simulink model "Compressor_MCU_Simulation_Architecture"  (R2018a)
settings: Solver=FixedStepDiscrete  StartTime=0.0  StopTime=30  FixedStep=TimeSteps.ModelStep  RelTol=1e-6
PreLoadFcn:
  | addpath('tools');
  | addpath('tools\Config_UI');
  | addpath('tools\support');
  | addpath('tools\FMIKit_for_Simulink');
  | addpath('tools\FMIKit_for_Simulink\slx');
  | addpath('tools\SpeedCommand');
  | addpath('tools\SpeedCommand\exe');
  | addpath('tools\SpeedCommand\view');
  | addpath('tools\MciAPI');
  | addpath('tools\MciAPI\exe');
  | addpath('tools\MciAPI\exe\enums');
  | addpath('tools\Read_PDB_File');
  | addpath('tools\Read_PDB_File\exe');
  | addpath('tools\PILComm');
  | addpath('tools\PILComm\exe');
  | 
  | addpath('exe');
  | addpath('source\c_code');
  | addpath('source\simulink\PlantModels\Sensor');
  | addpath('source\simulink\PlantModels\Rectifiers');
  | addpath('source\simulink\PlantModels\Motors\CIM');
  | addpath('source\simulink\PlantModels\Motors\BPM');
  | addpath('source\simulink\PlantModels\Motors\BPM\SFunctions\10k\Dyno');
  | addpath('source\simulink\PlantModels\Motors\BPM\SFunctions\10k\HA');
  | addpath('source\simulink\PlantModels\Motors\BPM\SFunctions\10k\VA_Agitation');
  | addpath('source\simulink\PlantModels\Motors\BPM\SFunctions\10k\VA_Spin');
  | addpath('source\simulink\PlantModels\Motors\BPM\SFunctions\16k\Dyno');
  | addpath('source\simulink\PlantModels\Motors\BPM\SFunctions\16k\HA');
  | addpath('source\simulink\PlantModels\Motors\BPM\SFunctions\16k\VA_Agitation');
  | addpath('source\simulink\PlantModels\Motors\BPM\SFunctions\16k\VA_Spin');
  | addpath('source\simulink\PlantModels\Inverter');
  | addpath('source\simulink\PlantModels\ADCModel');
  | 
  | 
  | addpath('exported_models');
  | clear all;
  | 
  | try
  | FMIKit.initialize()
  | catch
  | display('FMI Kit Initialization Skipped');
  | end
  | 
  | Sim_Arch_Config_UI_App;
PostLoadFcn:
  | myws = get_param(gcs, 'modelworkspace');
  | myws.clear;
  | clear myws;
  | evalin('base', 'recompile_mcu_sim_arch = 1;');
  | updateModelWS(gcs);
  | variant_adc_out_mode = 0;
InitFcn:
  | if (evalin('base', 'exist(''smlarch_need_reset'') == 1'))
  |     msgbox('Reload Variables before Running');
  |     set_param(gcs, 'SimulationCommand', 'stop');
  | end
  | BusInit;
  | if(  (exist('SimArchUID')) && (strcmp(SimArchUID, 'a') == 1)  )
  |     updateModelWS(gcs);
  | end
  | useModelWS(gcs);
  | Simulink.sdi.close;
model workspace (MAT data in the model file):
  DC_Bus.Const_Vbus = 325
  InputCircuit.R_line = 0.8
  InputCircuit.L_line = 5e-05
  InputCircuit.C_buscap = 0.00033
  InputCircuit.R_diode = 0.068
  InputCircuit.R_buscap = 0.603
  InputCircuit.V_knee = 0.75
  InputCircuit.G_off = 1.25e-08
  InputCircuit.L_pfc = 0.0097
  InputCircuit.R_pfc = 0.7
  InputCircuit.Vr = 230
  InputCircuit.Vdc_i = 300
  InputCircuit.freq = 50
  InputCircuit.C1 = -0.200926
  InputCircuit.C2 = 1.64303
  InputCircuit.Cvolt = 0.00738585
  InputCircuit.Vcc = 3.3
  InputCircuit.ADCBit = 12
  InputCircuit.PGA_Gain = 1
  Mechanical.belt_ratio = 10
  Mechanical.JDrum = 0.001
  Mechanical.damp = 0
  Mechanical.m_unb = 0
  Mechanical.r_unb = 0
  Mechanical.M_D = 1
  Mechanical.M = 0.2
  Mechanical.R_Drum = 0.254
  Mechanical.R_J = 0.05
  Mechanical.CF = 0
  Motor.Electrical.Rs_a_Ref = 1.7
  Motor.Electrical.Rs_b_Ref = 1.7
  Motor.Electrical.Rs_c_Ref = 1.7
  Motor.Electrical.p_Pole_Pairs = 3
  Motor.Electrical.PM_Flux_f01 = 0.1273
  Motor.Electrical.PM_Flux_f02 = 0
  Motor.Electrical.PM_Flux_f03 = 0
  Motor.Electrical.PM_Flux_f04 = 0
  Motor.Electrical.PM_Flux_f05 = 0
  Motor.Electrical.PM_Flux_f06 = 0
  Motor.Electrical.PM_Flux_f07 = 0
  Motor.Electrical.PM_Flux_f08 = 0
  Motor.Electrical.PM_Flux_f09 = 0
  Motor.Electrical.PM_Flux_f10 = 0
  Motor.Electrical.PM_Flux_f11 = 0
  Motor.Electrical.PM_Flux_f12 = 0
  Motor.Electrical.PM_Flux_f13 = 0
  Motor.Electrical.ajust = 1.57
  Motor.Electrical.alpha_s = 0.004
  Motor.Mechanical.Jrotor = 0.0002
  Motor.Mechanical.B = 0.002
  Motor.Mechanical.Jadd = 0
  Motor.Mechanical.Rs_Temperature_Ref = 22
  Motor.Mechanical.PM_Temperature_Ref = 22
  Motor.Mechanical.TR = 1
  Motor.Power_Loss.Rot_Loss_Flag = 0
  Motor.Power_Loss.Rot_Loss_Speed0 = 0
  Motor.Power_Loss.Rot_Loss_Speed1 = 500
  Motor.Power_Loss.Rot_Loss_Speed2 = 3000
  Motor.Power_Loss.Rot_Loss_Speed3 = 4000
  Motor.Power_Loss.Rot_Loss_Speed4 = 4000
  Motor.Power_Loss.Rot_Loss_Speed5 = 4000
  Motor.Power_Loss.Rot_Loss_Speed6 = 4000
  Motor.Power_Loss.Rot_Loss_Speed7 = 4000
  Motor.Power_Loss.Rot_Loss_Power0 = 0
  Motor.Power_Loss.Rot_Loss_Power1 = 0
  Motor.Power_Loss.Rot_Loss_Power2 = 0
  Motor.Power_Loss.Rot_Loss_Power3 = 0
  Motor.Power_Loss.Rot_Loss_Power4 = 0
  Motor.Power_Loss.Rot_Loss_Power5 = 0
  Motor.Power_Loss.Rot_Loss_Power6 = 0
  Motor.Power_Loss.Rot_Loss_Power7 = 0
  Motor.Inductance_Variation.Ld_a0 = 0.0205
  Motor.Inductance_Variation.Ld_a1 = 0.0205
  Motor.Inductance_Variation.Ld_a2 = 0.0205
  Motor.Inductance_Variation.Ld_a3 = 0.0205
  Motor.Inductance_Variation.Ld_a4 = 0.0205
  Motor.Inductance_Variation.Ld_a5 = 0.0205
  Motor.Inductance_Variation.Ld_a6 = 0.0205
  Motor.Inductance_Variation.Ld_a7 = 0.0205
  Motor.Inductance_Variation.Lq_b0 = 0.0205
  Motor.Inductance_Variation.Lq_b1 = 0.0205
  Motor.Inductance_Variation.Lq_b2 = 0.0205
  Motor.Inductance_Variation.Lq_b3 = 0.0205
  Motor.Inductance_Variation.Lq_b4 = 0.0205
  Motor.Inductance_Variation.Lq_b5 = 0.0205
  Motor.Inductance_Variation.Lq_b6 = 0.0205
  Motor.Inductance_Variation.Lq_b7 = 0.0205
  Motor.Inductance_Variation.I_pk0 = 0
  Motor.Inductance_Variation.I_pk1 = 1
  Motor.Inductance_Variation.I_pk2 = 2
  Motor.Inductance_Variation.I_pk3 = 3
  Motor.Inductance_Variation.I_pk4 = 4
  Motor.Inductance_Variation.I_pk5 = 5
  Motor.Inductance_Variation.I_pk6 = 6
  Motor.Inductance_Variation.I_pk7 = 7
  Paths.complete_file_R = 'settings\ParametersFiles\Rectifier_Parameters\HVPS_230VPFC\WindyStripH50_AC230VPFC.xml'
  Paths.complete_file_M = 'settings\ParametersFiles\Motor_Parameters\BPM\sBPM\BPM_RECHI_Heatpump.xml'
  Paths.complete_file_mc = 'settings\ParametersFiles\Mechanical_Parameters\HA\Mechanical_HA.xml'
  Paths.chosen_dir_M = 'settings\ParametersFiles\Motor_Parameters\BPM\sBPM'
  Paths.Setting_File_Path = 'C:\Data\Prj2021\Mcu_FOC_Control_Vcc_Dryer\exe\settingfile.bin'
  Paths.Root_Path = 'C:\Data\Prj2021\Mcu_FOC_Control_Vcc_Dryer\source'
  Paths.Object_Path = ''
  Thermal.Tstator = 22
  Thermal.Trotor = 22
  TimeSteps.ModelStep = 0.0001
  TimeSteps.InputCircuitStep = 0.0005
  Variant_Input_Circuit = 5
  Variant_Motor = 3
  Variant_Motor_Control = 1
  Variant_Sensor = 0
  config.MCI_Sampling_Frequency = 'Set'
  config.rect_flag = 0
  config.const_dcbus_flag = 1
  config.Root_Path_flag = 'Source Selected'
  config.Motor_Control_Source = 'Set'
  config.Control_Layer = 'SIL'
  config.Fast_ADC_Initialization_Flag = 'Set'
  config.Skip_Motor_Moving_Handler_Flag = 'Set'
  config.BoardVariant = 'AC230VPFC'
  config.MotorVariant = 'BPM_RECHI_Heatpump'
  config.MechanicalVariant = 'DynoLoad'
  config.Setting_File_Flag = 'Set'
undefined symbols (not defined in the file): sigbuilder_block, steps
libraries: pdb_libbrowser x6, mciapi_libbrowser x1
CloseFcn:
  | rmpath('support');
  | rmpath('Compile Scripts');
  | rmpath(genpath('Plant Models'));
  | rmpath(genpath('MciAPI'));
  | clc;
  | clear all;
settings Model: Creator=consul.marchionne  LastModifiedBy=BEATOA
settings DataIOCC: LimitDataPoints=on
settings OptimizationCC: LifeSpan=inf
settings DebuggingCC: SolverPrmCheckMsg=warning  SFUnexpectedBacktrackingDiag=warning  SFNoUnconditionalDefaultTransitionDiag=warning  SFExecutionAtInitializationDiag=none
settings HardwareCC: ProdBitPerPointer=32  ProdBitPerSizeT=32  ProdBitPerPtrDiffT=32  ProdLargestAtomicFloat=None  ProdIntDivRoundTo=Undefined  ProdEndianess=Unspecified  ProdWordSize=32  ProdHWDeviceType=32-bit Generic
settings ModelReferenceCC: UpdateModelReferenceTargets=IfOutOfDate  EnableRefExpFcnMdlSchedulingChecks=off  ModelReferenceNumInstancesAllowed=Single  ModelReferenceMinAlgLoopOccurrences=on  PropagateSignalLabelsOutOfModel=off
settings CodeAppCC: StateflowObjectComments=on
settings GRTTargetCC: TargetLangStandard=C89/C90 (ANSI)  GeneratePreprocessorConditionals=Disable all
settings ConfigComp: CovMetricSettings=dw  CovHtmlReporting=on  CovSaveCumulativeToWorkspaceVar=on  CovSaveSingleToWorkspaceVar=on  CovExternalEMLEnable=off  CovSFcnEnable=off

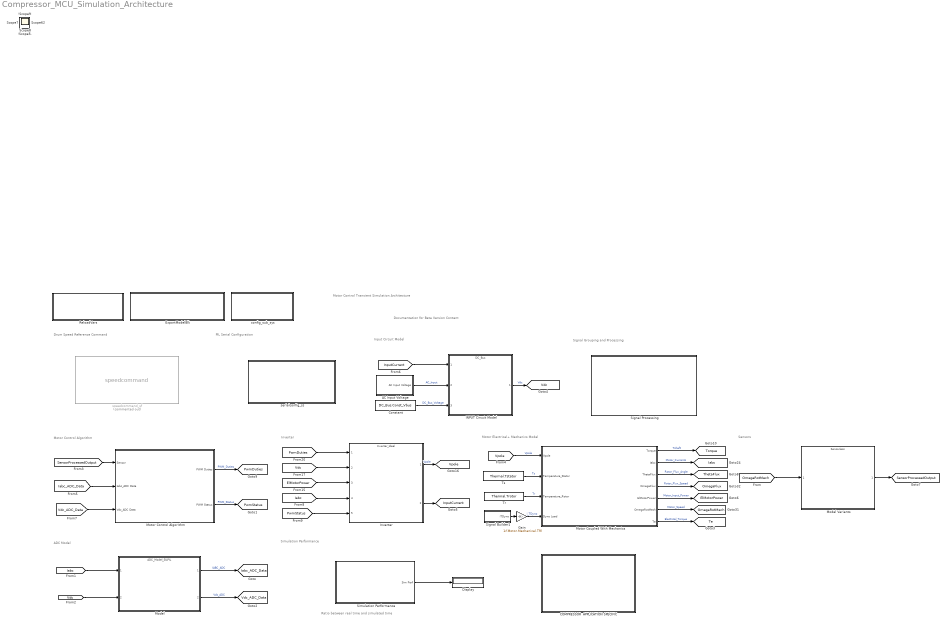
== system Compressor_MCU_Simulation_Architecture ==
  note: Motor Control Transient Simulation Architecture
  note: Input Circuit Model
  note: Simulation Performance
  note: Ratio between real time and simulated time
  note: ADC Model
  note: Motor Electrical+ Mechanics Model
  note: Inverter
  note: Signal Grouping and Processing
  note: PIL Serial Configuration
  note: Motor Control Algorithm
  note: Sensors
  note: Drum Speed Reference Command
  note: Documentation for Beta Version Content
  AC Input Voltage : Subsystem
  COMPRESSOR  APPLICATION SPECIFIC : Subsystem
  Constant : Constant  Value=DC_Bus.Const_Vbus
  Display : Display
  ExportModelBlk : Subsystem  LoadFcn=|  mask{model_name=}
      | msk = Simulink.Mask.get(gcb);
      | bHandle = msk.getDialogControl('Control2');
      | bHandle.Enabled = 'on';
      | clear msk;
      | clear bHandle;
      mask prompts: model_name "Model's export name (no extension)"
      mask DialogControl Control2 Prompt: Export
      mask DialogControl Control2 Callback:
      | save_system('MCU_Simulation_Architecture');
      | if (strcmp(get_param(gcb, 'model_name'),'') == 1)
      |     msgbox('Must give a name to the model');
      | else
      |     exportSimArch(get_param(gcb, 'model_name'));
      | end
      mask Display: disp('Export current configuration');
  Gain : Gain  Gain=1/(Motor.Mechanical.TR)
  INPUT Circuit Model : ModelReference  ModelNameDialog=DC_Bus.slx  SimulationMode=Normal  Variant=on  ModelReferenceVersion=1.7
      settings: AttributesFormatString=%<ActiveVariant>
  Inverter : ModelReference  ModelNameDialog=Inverter_Ideal.slx  SimulationMode=Normal  Variant=on  OverrideUsingVariant=Variant1  ModelReferenceVersion=1.14
      settings: AttributesFormatString=%<ActiveVariant>
  Model : ModelReference  ModelNameDialog=ADC_Model_SILPIL.slx  SimulationMode=Normal  ModelReferenceVersion=1.7
  Model Variants : ModelReference  ModelNameDialog=Sensorless.slx  SimulationMode=Normal  Variant=on  ModelReferenceVersion=1.8
      settings: AttributesFormatString=%<ActiveVariant>
  Motor Control Algorithm : Subsystem  SystemSampleTime=6.25e-5
  Motor Coupled With Mechanics : Subsystem  SystemSampleTime=0.000125
      settings: CopyFcn=|
      | blockname = gcb;
      |  linkstatus = lower(get_param(blockname,'LinkStatus'));
      | if strcmp(linkstatus,'resolved')
      |   set_param(gcb,'LinkStatus','none');
      | end
  ReloadVars : Subsystem
      settings: OpenFcn=|
      | evalin('base', 'clear smlarch_need_reset');
      | useModelWS(gcs);
      mask Display: disp('Reload Variables');
  Signal Builder1 : Subsystem  Tag=STV Subsys  LoadFcn=sigbuilder_block('load');  StartFcn=sigbuilder_block('start');  StopFcn=sigbuilder_block('stop');  ClipboardFcn=sigbuilder_block('clipboard');  mask(Sigbuilder block){tuvar=[0:10]}
      mask help: Simulink:masks:SigbuilderBlock_MD
      mask init:
      | if ~strcmp(get_param(bdroot(gcbh),'SimulationStatus'),'stopped') tuvar = sigbuilder_block('maskInit'); end
      settings: CopyFcn=sigbuilder_block('copy');  DeleteFcn=sigbuilder_block('delete');  ModelCloseFcn=sigbuilder_block('modelClose');  PreSaveFcn=sigbuilder_block('preSave');  PauseFcn=sigbuilder_block('pause');  ContinueFcn=sigbuilder_block('continue');  NameChangeFcn=sigbuilder_block('namechange');  OpenFcn=sigbuilder_block('open',[150 123 461.25 300 ]);  CloseFcn=sigbuilder_block('close');
      mask Display: plot(0, 0, 100, 100,[2, 2, 32, 32, 2], [68, 8, 8, 68, 68],[32, 2], [38, 38], [32, 19, 2],[53, 60, 44], [32, 17, 17, 2],[16, 16, 31, 31]);txt = getActiveGroup(gcbh);text(2, 100, txt,'verticalAlignment', 'top');
  Signal Processing : Subsystem
  Simulation Performance : Subsystem
  Tr : Constant  Value=Thermal.Trotor
  Ts : Constant  Value=Thermal.Tstator
  config_sub_sys : Subsystem  TreatAsAtomicUnit=on  mask{mcu_recompile=on}
      mask prompts: mcu_recompile "Recompile"
      mask Display:
      | if (strcmp(get_param(gcb, 'mcu_recompile'),'off') == 1)
      |     disp('Do not Recompile');
      | else
      |     disp('Recompile');
      | end
  serialconfig_ss : Subsystem  mask{comdevtype=RS232, com_port=COM4, baudrate=57600}
      mask prompts: comdevtype "COM Type"; com_port "COM Port"
      mask TypeOptions comdevtype: RS232 | SPI
      mask Callback comdevtype:
      | maskStr = get_param(gcb,'comdevtype');
      | if strcmp(maskStr,'SPI')
      |     assignin('base', 'VARIANT_PIL_COMM', 2);
      | else
      |     assignin('base', 'VARIANT_PIL_COMM', 1);
      | end
      | clear maskStr;
      mask TypeOptions com_port: COM3 | COM4
      mask TypeOptions baudrate: 2400 | 4800 | 9600 | 19200 | 28800 | 38400 | 57600 | 115200 | 230400
      mask DialogControl ParameterGroupVar Prompt: RS232 Settings
      mask DialogControl rfrsh_button Prompt: Refresh Ports
      mask DialogControl rfrsh_button Callback:
      | devices = winqueryreg('name', 'HKEY_LOCAL_MACHINE', 'HARDWARE\DEVICEMAP\SERIALCOMM');
      | if (isempty(devices))
      |     com{1} = 'NONE';
      | else
      |     com = cell(1, length(devices));
      |    % h = waitbar(0,'Scanning Serial Ports...','Name','Scanning Serial Ports...');
      |     for i = 1:length(devices)
      |         com{i} = winqueryreg('HKEY_LOCAL_MACHINE', 'HARDWARE\DEVICEMAP\SERIALCOMM', devices{i});
      |     %    waitbar(i/length(devices),h);
      |     end
      | end
      | 
      | msk = Simulink.Mask.get(gcb);
      | p = msk.Parameters;
      | p(2).TypeOptions = com;
      | clear msk;
      | clear p;
      | clear com;
      | clear devices;
      mask Display: disp('Serial Configuration');
  speedcommand_sf : S-Function  Commented=on  InitFcn=|  StopFcn=|  FunctionName=speedcommand  Parameters=steps, Variant_Motor_Control  SFunctionDeploymentMode=off  EnableBusSupport=off
      InitFcn=|
      | transmission = evalin('base','Motor.Mechanical.TR');
      | if isempty(get_param(gcb,'UserData'))
      | steps = [];
      | else
      |     ud = get_param(gcb,'UserData');
      |     [pts,steps] = GenPlotCmds(ud.table);
      |     for i = 1:size(steps,1)
      |         steps(i,1) = steps(i,1) * transmission;
      |         steps(i,2) = steps(i,2) * transmission;
      |     end
      | end
      | clear transmission;
      | clear i;
      | clear ud;
      StopFcn=|
      | clear steps;
      | clear pts;
      settings: OpenFcn=SpeedCommandView;
  Scope{,2..12} (12 alike) : Scope
  tag scope: ElMotorPower=global, Iabc=global, Iabc_ADC_Data=global, InputCurrent=global, OmegaFlux=global, OmegaRotMech=global, PwmDuties=global, PwmStatus=global, SensorProcessedOutput=global, Te=global, ThetaFlux=global, Torque=global, Vdc=global, Vdc_ADC_Data=global, Vpole=global
  wires:
  [OmegaRotMech] -> Model Variants/1
  Simulation Performance/1(Sim Perf) -> Display/1
  [Vpole] -> Motor Coupled With Mechanics/1(Vpole)  "Vpole"
  Motor Coupled With Mechanics/1(Torque) -> [Torque]  "Tshaft"
  Motor Coupled With Mechanics/2(Iabc) -> [Iabc]  "Motor_Currents"
  Motor Coupled With Mechanics/3(ThetaFlux) -> [ThetaFlux]  "Rotor_Flux_Angle"
  Motor Coupled With Mechanics/4(OmegaFlux) -> [OmegaFlux]  "Rotor_Flux_Speed"
  Motor Coupled With Mechanics/5(ElMotorPower) -> [ElMotorPower]  "Motor_Input_Power"
  Motor Coupled With Mechanics/6(OmegaRotMech) -> [OmegaRotMech]  "Motor_Speed"
  [PwmDuties] -> Inverter/1
  [Vdc] -> Inverter/2
  [ElMotorPower] -> Inverter/3
  [Iabc] -> Inverter/4
  Inverter/1 -> [Vpole]  "Vpole"
  Inverter/2 -> [InputCurrent]
  Motor Control Algorithm/1(PWM Duties) -> [PwmDuties]  "PWM_Duties"
  Motor Control Algorithm/2(PWM Status) -> [PwmStatus]  "PWM_Status"
  [SensorProcessedOutput] -> Motor Control Algorithm/1(Sensor)
  INPUT Circuit Model/1 -> [Vdc]  "Vdc"
  Constant/1 -> INPUT Circuit Model/3  "DC_Bus_Voltage"
  AC Input Voltage/1(AC Input Voltage) -> INPUT Circuit Model/2  "AC_Input"
  [InputCurrent] -> INPUT Circuit Model/1
  Model Variants/1 -> [SensorProcessedOutput]
  [PwmStatus] -> Inverter/5
  [Vdc] -> Model/2
  [Iabc] -> Model/1
  [Iabc_ADC_Data] -> Motor Control Algorithm/2(Iabc_ADC Data)
  Model/1 -> [Iabc_ADC_Data]  "IABC_ADC"
  Model/2 -> [Vdc_ADC_Data]  "Vdc_ADC"
  [Vdc_ADC_Data] -> Motor Control Algorithm/3(Vdc_ADC Data)
  Ts/1 -> Motor Coupled With Mechanics/2(Temperature_Stator)  "Ts"
  Tr/1 -> Motor Coupled With Mechanics/3(Temperature_Rotor)  "Tr"
  Gain/1 -> Motor Coupled With Mechanics/4(Dyno Load)  "i_TDyno"
  Signal Builder1/1(iTDyno) -> Gain/1
  Motor Coupled With Mechanics/7(Te) -> [Te]  "Electrical_Torque"

== system Compressor_MCU_Simulation_Architecture/AC Input Voltage ==
  Sine Wave : Sin  Amplitude=InputCircuit.Vr*sqrt(2)  Frequency=InputCircuit.freq*2*pi
  AC Input Voltage : Outport
  wires:
  Sine Wave/1 -> AC Input Voltage/1

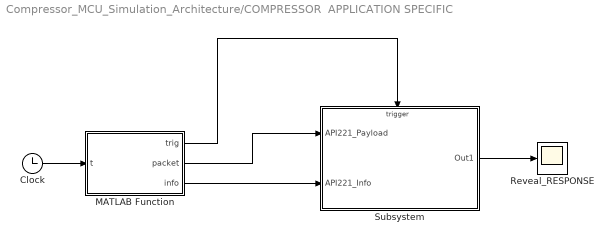
== system Compressor_MCU_Simulation_Architecture/COMPRESSOR  APPLICATION SPECIFIC ==
  Clock : Clock
  MATLAB Function : MATLAB Function  TreatAsAtomicUnit=on
  Reveal_RESPONSE : Scope
  Subsystem : Subsystem
  wires:
  MATLAB Function/1(trig) -> Subsystem/Trigger
  MATLAB Function/2(packet) -> Subsystem/1(API221_Payload)
  Clock/1 -> MATLAB Function/1(t)
  Subsystem/1(Out1) -> Reveal_RESPONSE/1
  MATLAB Function/3(info) -> Subsystem/2(API221_Info)

== system Compressor_MCU_Simulation_Architecture/ExportModelBlk ==

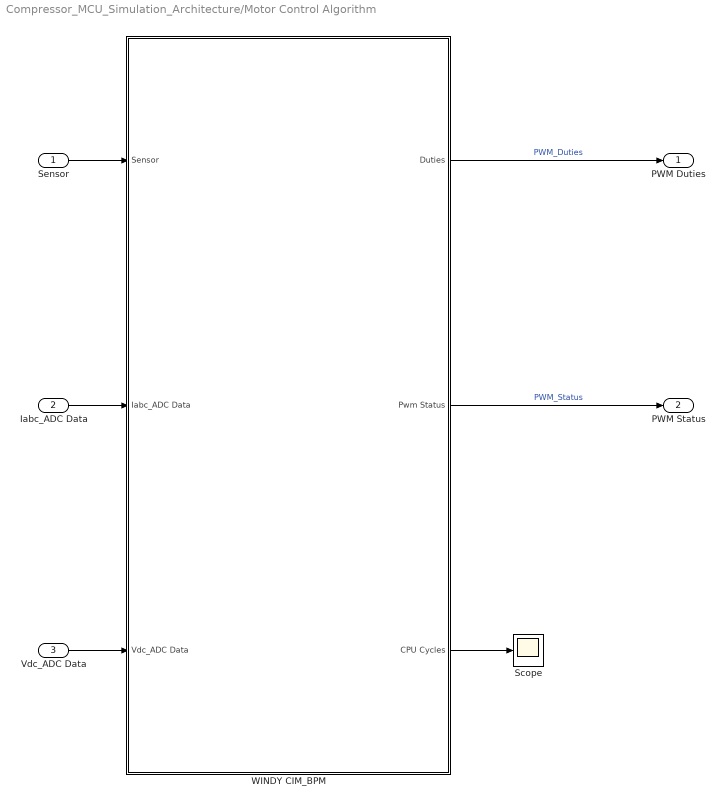
== system Compressor_MCU_Simulation_Architecture/Motor Control Algorithm ==
  Sensor : Inport
  Iabc_ADC Data : Inport  Port=2
  Vdc_ADC Data : Inport  Port=3
  Scope : Scope
  WINDY CIM_BPM : Subsystem  Variant=on
  PWM Duties : Outport
  PWM Status : Outport  Port=2
  wires:
  WINDY CIM_BPM/1(Duties) -> PWM Duties/1  "PWM_Duties"
  WINDY CIM_BPM/2(Pwm Status) -> PWM Status/1  "PWM_Status"
  Sensor/1 -> WINDY CIM_BPM/1(Sensor)
  Iabc_ADC Data/1 -> WINDY CIM_BPM/2(Iabc_ADC Data)
  Vdc_ADC Data/1 -> WINDY CIM_BPM/3(Vdc_ADC Data)
  WINDY CIM_BPM/3(CPU Cycles) -> Scope/1

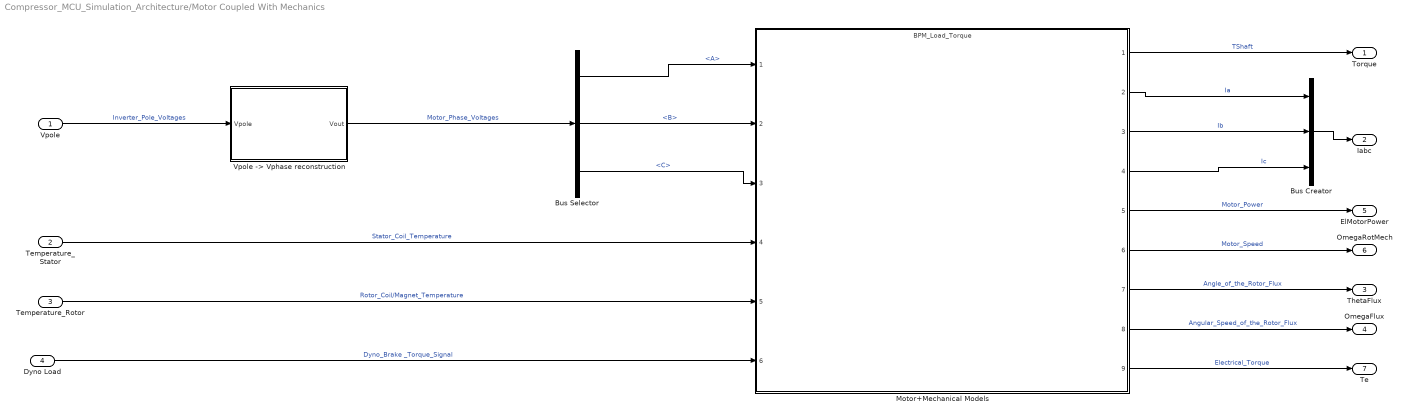
== system Compressor_MCU_Simulation_Architecture/Motor Coupled With Mechanics ==
  Vpole : Inport  OutDataTypeStr=Bus: XabcBus
  Temperature_Stator : Inport  Port=2
  Temperature_Rotor : Inport  Port=3
  Dyno Load : Inport  Port=4
  Bus Creator : BusCreator  Inputs=3
  Bus Selector : BusSelector  OutputSignals=A,B,C
  Motor+Mechanical Models : ModelReference  ModelNameDialog=BPM_Load_Torque.slx  SimulationMode=Normal  Variant=on  ModelReferenceVersion=1.264
      settings: AttributesFormatString=%<ActiveVariant>
  "Vpole -> Vphase reconstruction" : MATLAB Function  TreatAsAtomicUnit=on
  Torque : Outport
  Iabc : Outport  Port=2  OutDataTypeStr=Bus: XabcBus
  ThetaFlux : Outport  Port=3
  OmegaFlux : Outport  Port=4
  ElMotorPower : Outport  Port=5
  OmegaRotMech : Outport  Port=6
  Te : Outport  Port=7
  wires:
  Bus Creator/1 -> Iabc/1
  Vpole/1 -> "Vpole -> Vphase reconstruction"/1(Vpole)  "Inverter_Pole_Voltages"
  "Vpole -> Vphase reconstruction"/1(Vout) -> Bus Selector/1  "Motor_Phase_Voltages"
  Bus Selector/1 -> Motor+Mechanical Models/1  "<A>"
  Bus Selector/2 -> Motor+Mechanical Models/2  "<B>"
  Bus Selector/3 -> Motor+Mechanical Models/3  "<C>"
  Temperature_Stator/1 -> Motor+Mechanical Models/4  "Stator_Coil_Temperature"
  Temperature_Rotor/1 -> Motor+Mechanical Models/5  "Rotor_Coil/Magnet_Temperature"
  Motor+Mechanical Models/1 -> Torque/1  "TShaft"
  Motor+Mechanical Models/2 -> Bus Creator/1  "Ia"
  Motor+Mechanical Models/3 -> Bus Creator/2  "Ib"
  Motor+Mechanical Models/4 -> Bus Creator/3  "Ic"
  Motor+Mechanical Models/5 -> ElMotorPower/1  "Motor_Power"
  Motor+Mechanical Models/6 -> OmegaRotMech/1  "Motor_Speed"
  Motor+Mechanical Models/7 -> ThetaFlux/1  "Angle_of_the_Rotor_Flux"
  Dyno Load/1 -> Motor+Mechanical Models/6  "Dyno_Brake _Torque_Signal"
  Motor+Mechanical Models/8 -> OmegaFlux/1  "Angular_Speed_of_the_Rotor_Flux"
  Motor+Mechanical Models/9 -> Te/1  "Electrical_Torque"

== system Compressor_MCU_Simulation_Architecture/ReloadVars ==

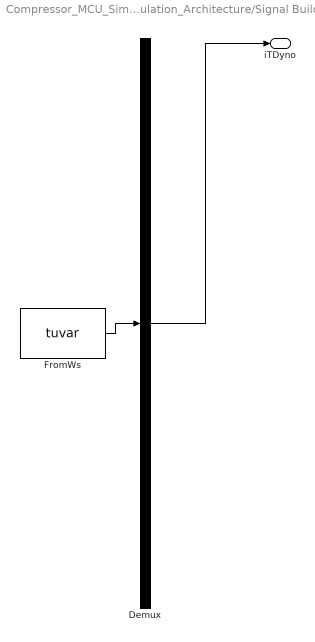
== system Compressor_MCU_Simulation_Architecture/Signal Builder1 ==
  Demux : Demux  Tag=STV Demux  Outputs=1
  FromWs : FromWorkspace  Tag=STV FromWs  VariableName=tuvar  SampleTime=0
      SigBuilderData=|
      | common.afterFinalStr = 'Extrapolate'
      | common.sampleTime = 0
      | dataSet.timeRange = [0 30]
      | dataSet.name = 'Dyno_Load_Profile'
      | sbobj.Groups.Name = 'Dyno_Load_Profile'
      | sbobj.Groups.Signals.Name = 'iTDyno'
      | sbobj.Groups.Signals.XData = [0 0.8 4 20 28 30]
      | sbobj.Groups.Signals.YData = [0 0 0 0 0 0]
      | sbobj.Groups.TimeRange = [0 30]
  iTDyno : Outport  Tag=STV Outport
  wires:
  Demux/1 -> iTDyno/1
  FromWs/1 -> Demux/1

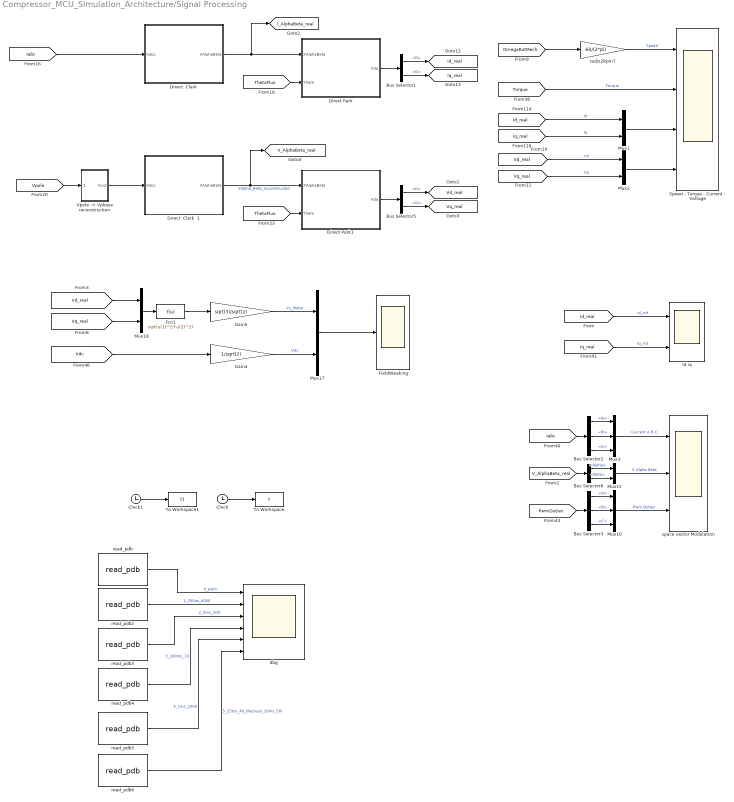
== system Compressor_MCU_Simulation_Architecture/Signal Processing ==
  Bus Selector1 : BusSelector  OutputSignals=D,Q
  Bus Selector2 : BusSelector  OutputSignals=Ia,Ib,Ic
  Bus Selector3 : BusSelector  OutputSignals=A,B,C
  Bus Selector5 : BusSelector  OutputSignals=D,Q
  Bus Selector6 : BusSelector  OutputSignals=Alpha,Beta
  Clock : Clock
  Clock1 : Clock
  "Direct  Clark  " : MATLAB Function  TreatAsAtomicUnit=on  SystemSampleTime=SystemSampleTime  mask{SystemSampleTime=-1}
      mask prompts: SystemSampleTime "Simulink:blkprm_prompts:AllBlksSampleTime"
  Direct  Clark  1 : MATLAB Function  TreatAsAtomicUnit=on  SystemSampleTime=SystemSampleTime  mask{SystemSampleTime=-1}
      mask prompts: SystemSampleTime "Simulink:blkprm_prompts:AllBlksSampleTime"
  Direct Park : MATLAB Function  TreatAsAtomicUnit=on  SystemSampleTime=SystemSampleTime  mask{SystemSampleTime=-1}
      mask prompts: SystemSampleTime "Simulink:blkprm_prompts:AllBlksSampleTime"
  Direct Park1 : MATLAB Function  TreatAsAtomicUnit=on  SystemSampleTime=SystemSampleTime  mask{SystemSampleTime=-1}
      mask prompts: SystemSampleTime "Simulink:blkprm_prompts:AllBlksSampleTime"
  Fcn1 : Fcn  Expr=sqrt(u(1)^2+u(2)^2)
  "FieldWeaking " : Scope
  Gain4 : Gain  Gain=1/sqrt(2)
  Gain5 : Gain  Gain=sqrt(3)/sqrt(2)
  Id iq : Scope  NumInputPorts=2
  Mux{1..2,15,17..18} (5 alike) : Mux  Inputs=2
  Mux10 : Mux  Inputs=3
  Mux3 : Mux  Inputs=3
  Speed - Torque - Current - Voltage : Scope  NumInputPorts=4
  To Workspace : ToWorkspace  VariableName=t  SampleTime=-1
      settings: Save2DSignal=2-D array (concatenate along first dimension)
  To Workspace1 : ToWorkspace  VariableName=t1  SampleTime=-1
      settings: Save2DSignal=2-D array (concatenate along first dimension)
  "Vpole -> Vphase reconstruction" : MATLAB Function  TreatAsAtomicUnit=on
  dbg : Scope  NumInputPorts=6
  rad/s2Rpm7 : Gain  Gain=60/(2*pi)
  read_pdb : pdb_libbrowser/read_pdb  vstring=dbg_scheduler_0
      settings: SourceProductName=Sim Arch
  read_pdb2 : pdb_libbrowser/read_pdb  vstring=dbg_scheduler_1
      settings: SourceProductName=Sim Arch
  read_pdb3 : pdb_libbrowser/read_pdb  vstring=dbg_scheduler_2
      settings: SourceProductName=Sim Arch
  read_pdb4 : pdb_libbrowser/read_pdb  vstring=dbg_scheduler_3
      settings: SourceProductName=Sim Arch
  read_pdb5 : pdb_libbrowser/read_pdb  vstring=dbg_scheduler_4
      settings: SourceProductName=Sim Arch
  read_pdb6 : pdb_libbrowser/read_pdb  vstring=dbg_scheduler_5
      settings: SourceProductName=Sim Arch
  space vector Modulation : Scope  NumInputPorts=3
  tag scope: I_AlphaBeta_real=global, Id_real=global, Iq_real=global, V_AlphaBeta_real=global, Vd_real=global, Vq_real=global
  wires:
  [OmegaRotMech] -> rad/s2Rpm7/1
  rad/s2Rpm7/1 -> Speed - Torque - Current - Voltage/1  "Speed"
  [Vq_real] -> Mux2/2  "Vq"
  [Id_real] -> Mux1/1  "Id"
  [Iabc] -> "Direct  Clark  "/1(Xabc)
  Direct Park/1(Xdq) -> Bus Selector1/1
  Bus Selector1/1 -> [Id_real]  "<D>"
  Bus Selector1/2 -> [Iq_real]  "<Q>"
  Fcn1/1 -> Gain5/1
  Mux18/1 -> Fcn1/1
  [Vd_real] -> Mux18/1
  [Vq_real] -> Mux18/2
  Mux17/1 -> "FieldWeaking "/1
  [Vdc] -> Gain4/1
  Bus Selector3/1 -> Mux10/1  "<A>"
  Bus Selector3/2 -> Mux10/2  "<B>"
  Bus Selector3/3 -> Mux10/3  "<C>"
  Mux10/1 -> space vector Modulation/3  "Pwm Duties"
  Bus Selector2/1 -> Mux3/1  "<Ia>"
  Bus Selector2/2 -> Mux3/2  "<Ib>"
  Bus Selector2/3 -> Mux3/3  "<Ic>"
  [Iabc] -> Bus Selector2/1
  [PwmDuties] -> Bus Selector3/1
  "Direct  Clark  "/1(XAlphaBeta) -> [I_AlphaBeta_real], Direct Park/1(XAlphaBeta)
  Clock/1 -> To Workspace/1
  Clock1/1 -> To Workspace1/1
  [Id_real] -> Id iq/1  "Id_rot"
  [Iq_real] -> Id iq/2  "Iq_rot"
  Gain4/1 -> Mux17/2  "Vdc"
  Gain5/1 -> Mux17/1  "Vs_Motor"
  Mux3/1 -> space vector Modulation/1  "Current A B C"
  [ThetaFlux] -> Direct Park/2(Theta)
  "Vpole -> Vphase reconstruction"/1(Vout) -> Direct  Clark  1/1(Xabc)
  [Vpole] -> "Vpole -> Vphase reconstruction"/1(Vpole)
  Direct  Clark  1/1(XAlphaBeta) -> Direct Park1/1(XAlphaBeta), [V_AlphaBeta_real]  "Valpha_Beta_reconstructed"
  [V_AlphaBeta_real] -> Bus Selector6/1
  Bus Selector6/1 -> Mux15/1  "<Alpha>"
  Bus Selector6/2 -> Mux15/2  "<Beta>"
  Mux15/1 -> space vector Modulation/2  "V Alpha Beta"
  Bus Selector5/2 -> [Vq_real]  "<Q>"
  Bus Selector5/1 -> [Vd_real]  "<D>"
  [ThetaFlux] -> Direct Park1/2(Theta)
  Direct Park1/1(Xdq) -> Bus Selector5/1
  [Iq_real] -> Mux1/2  "Iq"
  [Vd_real] -> Mux2/1  "Vd"
  [Torque] -> Speed - Torque - Current - Voltage/2  "Torque"
  Mux2/1 -> Speed - Torque - Current - Voltage/4
  Mux1/1 -> Speed - Torque - Current - Voltage/3
  read_pdb4/1 -> dbg/4  "3_100ms_10"
  read_pdb6/1 -> dbg/6  "5_25ms_40_(Nucleus_20ms_50)"
  read_pdb3/1 -> dbg/3  "2_5ms_200"
  read_pdb5/1 -> dbg/5  "4_1ms_1000"
  read_pdb2/1 -> dbg/2  "1_250us_4000"
  read_pdb/1 -> dbg/1  "0_pwm"

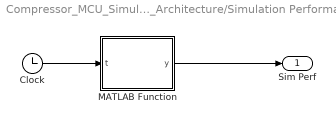
== system Compressor_MCU_Simulation_Architecture/Simulation Performance ==
  Clock : Clock
  MATLAB Function : MATLAB Function  TreatAsAtomicUnit=on
  Sim Perf : Outport
  wires:
  MATLAB Function/1(y) -> Sim Perf/1
  Clock/1 -> MATLAB Function/1(t)

== system Compressor_MCU_Simulation_Architecture/config_sub_sys ==

== system Compressor_MCU_Simulation_Architecture/serialconfig_ss ==

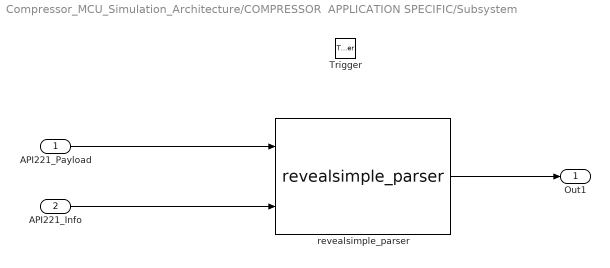
== system Compressor_MCU_Simulation_Architecture/COMPRESSOR  APPLICATION SPECIFIC/Subsystem ==
  API221_Payload : Inport
  API221_Info : Inport  Port=2
  Trigger : TriggerPort  VariantControl=Variant  PortDimensions=1
  revealsimple_parser : mciapi_libbrowser/revealsimple_parser  SFunctionModules=''
      settings: SourceProductName=Sim Arch
  Out1 : Outport
  wires:
  revealsimple_parser/1 -> Out1/1
  API221_Payload/1 -> revealsimple_parser/1
  API221_Info/1 -> revealsimple_parser/2

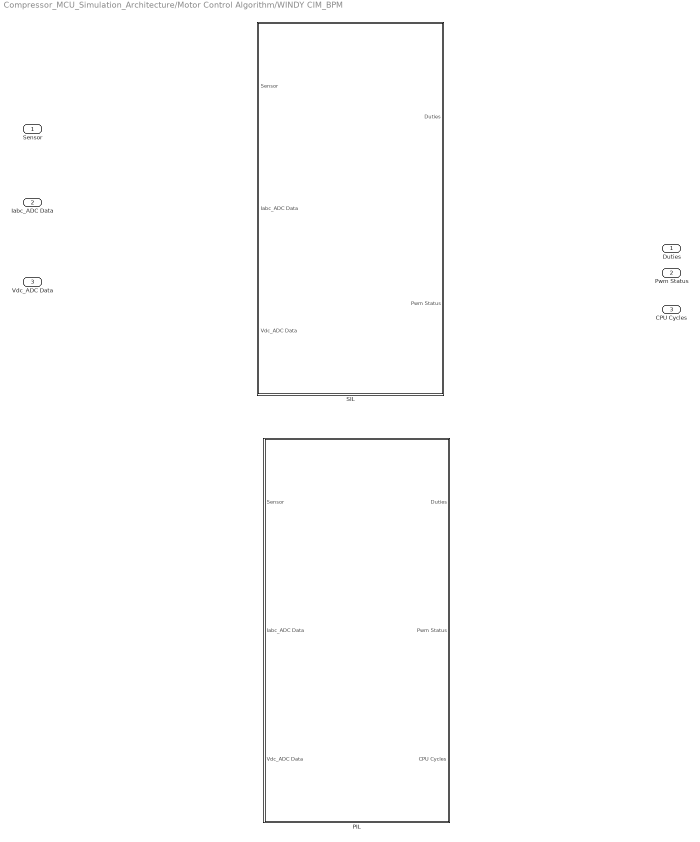
== system Compressor_MCU_Simulation_Architecture/Motor Control Algorithm/WINDY CIM_BPM ==
  Sensor : Inport
  Iabc_ADC Data : Inport  Port=2
  Vdc_ADC Data : Inport  Port=3
  PIL : Subsystem  InitFcn=|  VariantControl=Variant_Motor_Control==2
      | Control_Layer=evalin('base','config.Control_Layer');
      | 
      | switch Control_Layer
      |    case 'MCI'
      | 
      |      Compile_Link_MCI(config.Root_Path_flag, Paths.Root_Path, config.Motor, Paths.Object_Path)
      | 
      | case 'MCU'
      |    
      |      Compile_Link_MCU(config.Root_Path_flag, Paths.Root_Path, config.Motor, Paths.Object_Path)
      | end
      | 
      | clear Control_Layer;
  SIL : Subsystem  VariantControl=Variant_Motor_Control==1
  Duties : Outport
  Pwm Status : Outport  Port=2
  CPU Cycles : Outport  Port=3

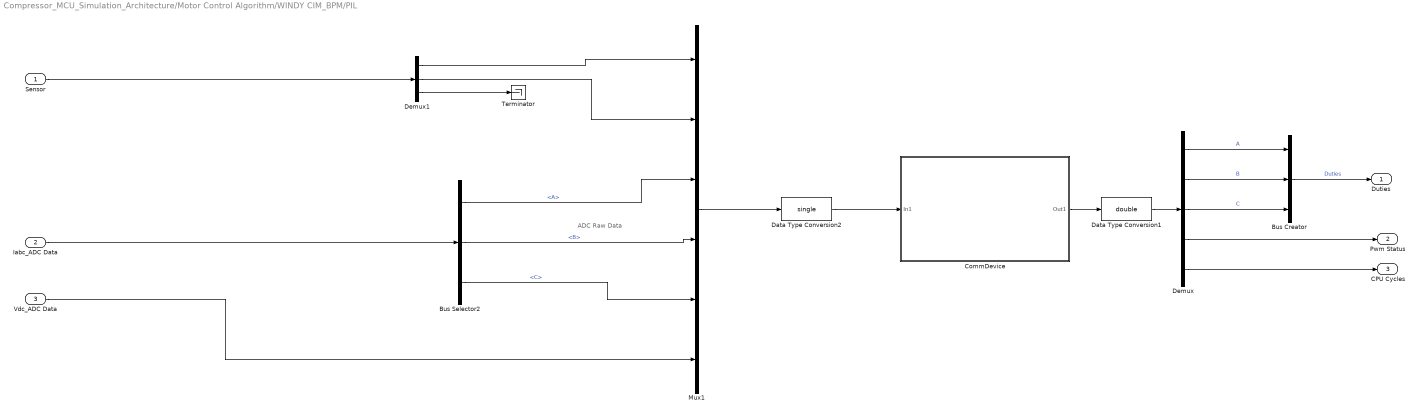
== system Compressor_MCU_Simulation_Architecture/Motor Control Algorithm/WINDY CIM_BPM/PIL ==
  note: ADC Raw Data
  Sensor : Inport
  Iabc_ADC Data : Inport  Port=2
  Vdc_ADC Data : Inport  Port=3
  Bus Creator : BusCreator  Inputs=3
  Bus Selector2 : BusSelector  OutputSignals=A,B,C
  CommDevice : Subsystem  Variant=on  VariantControl=Variant1
  Data Type Conversion1 : DataTypeConversion  OutDataTypeStr=double
  Data Type Conversion2 : DataTypeConversion  OutDataTypeStr=single
  Demux : Demux  Outputs=5
  Demux1 : Demux  Outputs=3
  Mux1 : Mux  Inputs=6
  Terminator : Terminator
  Duties : Outport
  Pwm Status : Outport  Port=2
  CPU Cycles : Outport  Port=3
  wires:
  Bus Creator/1 -> Duties/1  "Duties"
  Bus Selector2/2 -> Mux1/4  "<B>"
  Bus Selector2/1 -> Mux1/3  "<A>"
  Bus Selector2/3 -> Mux1/5  "<C>"
  Vdc_ADC Data/1 -> Mux1/6
  Iabc_ADC Data/1 -> Bus Selector2/1
  Sensor/1 -> Demux1/1
  Demux1/3 -> Terminator/1
  Demux1/1 -> Mux1/1
  Demux1/2 -> Mux1/2
  Mux1/1 -> Data Type Conversion2/1
  Data Type Conversion2/1 -> CommDevice/1("In1 ")
  Data Type Conversion1/1 -> Demux/1
  Demux/4 -> Pwm Status/1
  Demux/1 -> Bus Creator/1  "A"
  Demux/2 -> Bus Creator/2  "B"
  Demux/3 -> Bus Creator/3  "C"
  CommDevice/1(" Out1") -> Data Type Conversion1/1
  Demux/5 -> CPU Cycles/1

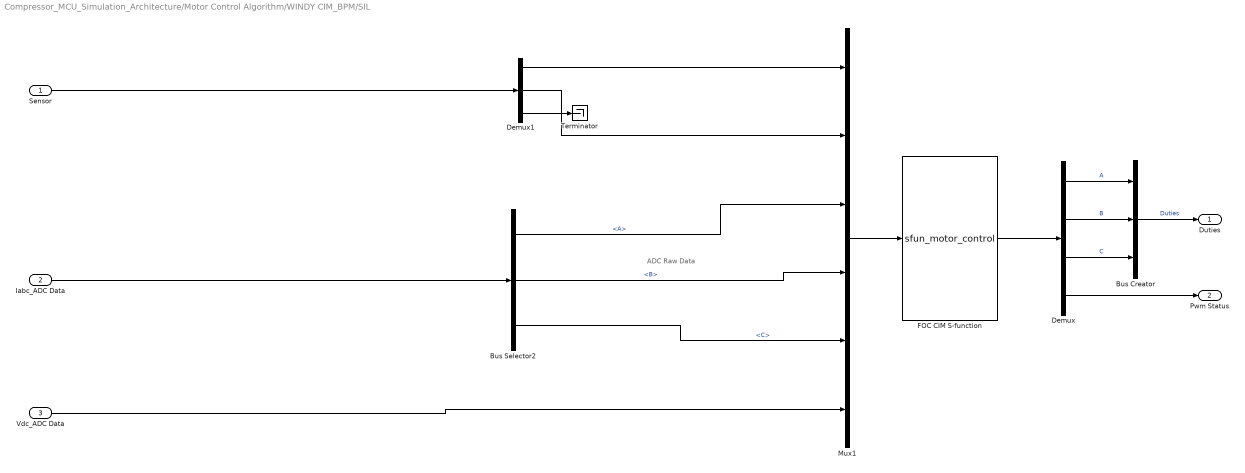
== system Compressor_MCU_Simulation_Architecture/Motor Control Algorithm/WINDY CIM_BPM/SIL ==
  note: ADC Raw Data
  Sensor : Inport
  Iabc_ADC Data : Inport  Port=2
  Vdc_ADC Data : Inport  Port=3
  Bus Creator : BusCreator  Inputs=3
  Bus Selector2 : BusSelector  OutputSignals=A,B,C
  Demux : Demux
  Demux1 : Demux  Outputs=3
  "FOC CIM S-function " : S-Function  InitFcn=|  StopFcn=clear CompileStruct;  FunctionName=sfun_motor_control  Parameters=TimeSteps.ModelStep,Paths.Setting_File_Path  SFunctionDeploymentMode=off  EnableBusSupport=off
      | clear mex;
      | CompileStruct.Root_Path_flag=config.Root_Path_flag;
      | CompileStruct.Root_Path=Paths.Root_Path;
      | CompileStruct.Object_Path=Paths.Object_Path;
      | CompileStruct.Fast_ADC_Initialization_Flag=config.Fast_ADC_Initialization_Flag;
      | CompileStruct.Skip_Motor_Moving_Handler_Flag=config.Skip_Motor_Moving_Handler_Flag;
      | CompileStruct.Setting_File_Flag=config.Setting_File_Flag;
      | 
      | if ( (strcmp(get_param('MCU_Simulation_Architecture/config_sub_sys', 'mcu_recompile'), 'on') == 1) || (exist('SimArchUID')==0) || ( strcmp(SimArchUID, 'a') == 0 ) )
      |     Compile_Link_MCU(CompileStruct);
      |     assignin('base', 'SimArchUID', 'a');
      | end
  Mux1 : Mux  Inputs=6
  Terminator : Terminator
  Duties : Outport
  Pwm Status : Outport  Port=2
  wires:
  Bus Selector2/2 -> Mux1/4  "<B>"
  "FOC CIM S-function "/1 -> Demux/1
  Bus Selector2/1 -> Mux1/3  "<A>"
  Bus Selector2/3 -> Mux1/5  "<C>"
  Vdc_ADC Data/1 -> Mux1/6
  Bus Creator/1 -> Duties/1  "Duties"
  Iabc_ADC Data/1 -> Bus Selector2/1
  Mux1/1 -> "FOC CIM S-function "/1
  Demux1/1 -> Mux1/1
  Demux1/2 -> Mux1/2
  Demux1/3 -> Terminator/1
  Sensor/1 -> Demux1/1
  Demux/1 -> Bus Creator/1  "A"
  Demux/2 -> Bus Creator/2  "B"
  Demux/3 -> Bus Creator/3  "C"
  Demux/4 -> Pwm Status/1

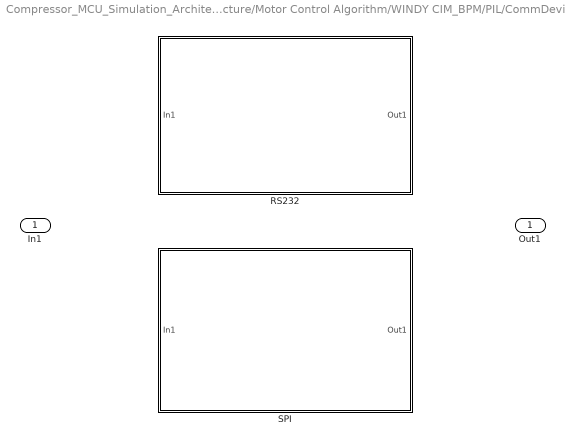
== system Compressor_MCU_Simulation_Architecture/Motor Control Algorithm/WINDY CIM_BPM/PIL/CommDevice ==
  "In1 " : Inport
  RS232 : Subsystem  VariantControl=VARIANT_PIL_COMM == 1
  SPI : Subsystem  VariantControl=VARIANT_PIL_COMM == 2
  " Out1" : Outport

== system Compressor_MCU_Simulation_Architecture/Motor Control Algorithm/WINDY CIM_BPM/PIL/CommDevice/RS232 ==
  In1 : Inport
  PIL_Comm : S-Function  InitFcn=|  FunctionName=serial_sf  Parameters=get_param([bdroot '/serialconfig_ss'], 'com_port'), get_param([bdroot '/serialconfig_ss'], 'baudrate'), steps  SFunctionDeploymentMode=off  EnableBusSupport=off
      | transmission = evalin('base','Motor.Mechanical.TR');
      | spd_blk = [bdroot '/speedcommand_sf']
      | if isempty(get_param(spd_blk,'UserData'))
      | steps = [];
      | else
      |     ud = get_param(spd_blk,'UserData');
      |     [pts,steps] = GenPlotCmds(ud.table);
      |     for i = 1:size(steps,1)
      |         steps(i,1) = steps(i,1) * transmission;
      |         steps(i,2) = steps(i,2) * transmission;
      |     end
      | end
      mask Display:
      | port_label('input', 1, 'Sim Inputs')
      | port_label('output', 1, 'Sim Outputs')
  Out1 : Outport
  wires:
  PIL_Comm/1 -> Out1/1
  In1/1 -> PIL_Comm/1

== system Compressor_MCU_Simulation_Architecture/Motor Control Algorithm/WINDY CIM_BPM/PIL/CommDevice/SPI ==
  "In1 " : Inport
  S-Function : S-Function  InitFcn=|  FunctionName=cheetah_sf  Parameters=steps  SFunctionDeploymentMode=off  EnableBusSupport=off
      | transmission = evalin('base','Motor.Mechanical.TR');
      | spd_blk = [bdroot '/speedcommand_sf']
      | if isempty(get_param(spd_blk,'UserData'))
      | steps = [];
      | else
      |     ud = get_param(spd_blk,'UserData');
      |     [pts,steps] = GenPlotCmds(ud.table);
      |     for i = 1:size(steps,1)
      |         steps(i,1) = steps(i,1) * transmission;
      |         steps(i,2) = steps(i,2) * transmission;
      |     end
      | end
  " Out1" : Outport
  wires:
  "In1 "/1 -> S-Function/1
  S-Function/1 -> " Out1"/1

== matlab function Compressor_MCU_Simulation_Architecture/Signal Processing/Direct  Clark  1 ==
  data: XAlphaBeta output Bus: XAlphaBetaBus; Xabc input Bus: XabcBus
function XAlphaBeta = DirectClark(Xabc)

XAlphaBeta.Alpha = Xabc.A;
XAlphaBeta.Beta =  sqrt(3)/3*(Xabc.A+2*Xabc.B);

== matlab function Compressor_MCU_Simulation_Architecture/Signal Processing/Direct  Clark   ==
  data: XAlphaBeta output Bus: XAlphaBetaBus; Xabc input Bus: XabcBus
function XAlphaBeta = DirectClark(Xabc)

XAlphaBeta.Alpha = Xabc.A;
XAlphaBeta.Beta =  sqrt(3)/3*(Xabc.A+2*Xabc.B);

== matlab function Compressor_MCU_Simulation_Architecture/Motor Coupled With Mechanics/Vpole -> Vphase reconstruction ==
  data: Vpole input Bus: XabcBus size=1; Vout output Bus: XabcBus
function Vout   = Vrec2(Vpole)

Va = Vpole.A;
Vb = Vpole.B;
Vc = Vpole.C;

Vn = (Va + Vb + Vc)/3;

Vphase.A = Va - Vn;
Vphase.B = Vb - Vn;
Vphase.C = Vc - Vn;

Vline.A = Va - Vb;  % Vab
Vline.B = Vb - Vc;  % Vbc
Vline.C = Vc - Va;  % Vca

Vout = Vphase;
end

== matlab function Compressor_MCU_Simulation_Architecture/COMPRESSOR  APPLICATION SPECIFIC/MATLAB Function ==
  data: trig output int32; packet output uint8; t input; info output
function [trig, packet, info]  = fcn(t)
packet = uint8(zeros(10,1));
persistent t_old;
if isempty(t_old)
    t_old = int32(0);
end

trig = int32(0);
server_motor = 0;
api_id = 221;
op_code_keep_run = 3; % Keep Running
op_code_stop = 4;  % Stop
op_code_run = 5; % Command Run
size = 0;
op_code = 0;

% trigger generation
t_round = int32(t);
if not(t_round == t_old) 
    if (t>4.4 && t<5.4)
        trig = int32(1);
        
        velocity = 4100;
        acceleration = 2800;
        op_code = op_code_run;
        packet_payload = uint8([server_motor; api221_format(velocity); api221_format(acceleration)]);
        size = 5;

        packet(1:length(packet_payload)) = packet_payload;
    end
    
    if (t>7.4 && t<8.4)
        trig = int32(1);
        
        op_code = op_code_keep_run;        
        packet_payload = uint8([server_motor]);
        size = 1;

        packet(1:length(packet_payload)) = packet_payload;
    end
    
    if (t>12.4 && t<13.4)
        trig = int32(1);

        velocity = 2100;
        acceleration = 1500;
        op_code = op_code_run;
        packet_payload = uint8([server_motor; api221_format(velocity); api221_format(acceleration)]);
        size = 5;

        packet(1:length(packet_payload)) = packet_payload;
    end

    if (t>17.4 && t<18.4)
        trig = int32(1);

        op_code = op_code_keep_run;        
        packet_payload = uint8([server_motor]);
        size = 1;

        packet(1:length(packet_payload)) = packet_payload;
    end
    
    if (t>22.4 && t<23.4)
        trig = int32(1);
        
        op_code = op_code_keep_run;        
        packet_payload = uint8([server_motor]);
        size = 1;
        
        packet(1:length(packet_payload)) = packet_payload;
    end
    
    if (t>26.4 && t<27.4)
        trig = int32(1);

        acceleration = 1000;
        op_code = op_code_stop; 
        packet_payload = uint8([server_motor; api221_format(acceleration)]);
        size = 3;
        
        packet(1:length(packet_payload)) = packet_payload;
    end


    
end

t_old = t_round;


destination = 0;
node_id = 1;
sdu_length = size + 2 ;
sap = 4;
cmd_fb = 0;
frag = 0;
mmp = 0;

info = uint8([destination; node_id; sdu_length; sap; api_id; op_code; cmd_fb; frag; mmp; size]);

end

function converted = api221_format(value)

converted = [fix(value/256) ; rem(value,256)];

end
% function [trig,packet]  = fcn(t)
% server_motor = 0;
% api = 221;
% op_code_keep_run = 3; % Keep Running
% op_code_stop = 4;  % Stop
% op_code_run = 5; % Command Run
% 
% trig = int32(0);
% packet = uint8([0; 0; 0; 0; 0; 0; 0; 0; 0; 0]);
% 
% if (t > 1) && (t<2)
%     trig = int32(1);    
% elseif (t>=5) && (t<6)
%     trig = int32(1);
% elseif (t>=10) && (t<11)
%     trig = int32(1);
% elseif (t>=15) && (t<16)
%     trig = int32(1);
% elseif (t>=20) && (t<21)
%     trig = int32(1);    
% elseif (t>=24) && (t<25)
%     trig = int32(1);
% end
% 
% 
% if (t<4.5)
%     velocity = 4100;
%     acceleration = 2800;
%     packet = uint8([api; op_code_run; server_motor; fix(velocity/256) ; rem(velocity,256); fix(acceleration/256) ; rem(acceleration,256); 0; 0; 0]);
% elseif (t<7)
%     packet = uint8([api; op_code_keep_run; server_motor; 0; 0; 0; 0; 0; 0; 0]);
% elseif (t<12)
%     velocity = 2100;
%     acceleration = 1500;
%     packet = uint8([api; op_code_run; server_motor; fix(velocity/256) ; rem(velocity,256); fix(acceleration/256) ; rem(acceleration,256); 0; 0; 0]);
% elseif (t<17)
%     packet = uint8([api; op_code_keep_run; server_motor; 0; 0; 0; 0; 0; 0; 0]);
% elseif (t<22)
%     packet = uint8([api; op_code_keep_run; server_motor; 0; 0; 0; 0; 0; 0; 0]);
% elseif (t<26)
%     acceleration = 1000;
%     packet = uint8([api; op_code_stop; server_motor; fix(acceleration/256) ; rem(acceleration,256); 0; 0; 0; 0; 0]);
% end
% %     speed = 0;
% % elseif (t>=11) && (t<16)
% %     speed = 3200;
% % end
% 
%

== matlab function Compressor_MCU_Simulation_Architecture/Simulation Performance/MATLAB Function ==
  data: t input; y output
function y = fcn(t)

persistent t_elaps tval sim_steps t_start t_end
coder.extrinsic('toc') 
coder.extrinsic('tic')
steps_start = 100;%10000;
steps_end = 500;%50000;

if isempty(tval)
    sim_steps = 0;
    tval = uint64(0);
    t_elaps = 0;
    t_start = 0;
    t_end = 0;
end
    
sim_steps = sim_steps +1;

if (sim_steps == steps_start)
    tval = tic;
    t_start = t;
     
end
if (sim_steps == steps_end)
    t_elaps = toc(tval);
    t_end = t;
end
 
if (t_elaps == 0)
    y = 0;
else
    y = t_elaps/(t_end-t_start);
 end

== matlab function Compressor_MCU_Simulation_Architecture/Signal Processing/Direct Park ==
  data: XAlphaBeta input Bus: XAlphaBetaBus; Xdq output Bus: XdqBus; Theta input
function Xdq = DirectPark(XAlphaBeta,Theta)

Xdq.D  =  XAlphaBeta.Alpha*cos(Theta) + XAlphaBeta.Beta*sin(Theta);
Xdq.Q  = -XAlphaBeta.Alpha*sin(Theta) + XAlphaBeta.Beta*cos(Theta);

== matlab function Compressor_MCU_Simulation_Architecture/Signal Processing/Direct Park1 ==
  data: XAlphaBeta input Bus: XAlphaBetaBus; Xdq output Bus: XdqBus; Theta input
function Xdq = DirectPark(XAlphaBeta,Theta)

Xdq.D  =  XAlphaBeta.Alpha*cos(Theta) + XAlphaBeta.Beta*sin(Theta);
Xdq.Q  = -XAlphaBeta.Alpha*sin(Theta) + XAlphaBeta.Beta*cos(Theta);

== matlab function Compressor_MCU_Simulation_Architecture/Signal Processing/Vpole -> Vphase reconstruction ==
  data: Vpole input Bus: XabcBus size=1; Vout output Bus: XabcBus
function Vout   = Vrec2(Vpole)

Va = Vpole.A;
Vb = Vpole.B;
Vc = Vpole.C;

Vn = (Va + Vb + Vc)/3;

Vphase.A = Va - Vn;
Vphase.B = Vb - Vn;
Vphase.C = Vc - Vn;

Vline.A = Va - Vb;  % Vab
Vline.B = Vb - Vc;  % Vbc
Vline.C = Vc - Va;  % Vca

Vout = Vphase;
end
